simulink model "MdBsyClear4s"  (R2018b)
settings: Solver=FixedStepDiscrete  StartTime=0.0  StopTime=10.0  FixedStep=0.01  RelTol=1e-3
undefined symbols (not defined in the file or in its folder): ClearBit, IsStBsy32_Clear
settings Model: ModifiedHistory=2023.8.1 V2.0.0 CR401790 增加模式21-26  Creator=sn2xws  LastModifiedBy=sn2xws
settings DataIOCC: SaveFormat=StructureWithTime
settings OptimizationCC: DefaultParameterBehavior=Inlined  EnhancedBackFolding=on  PassReuseOutputArgsAs=Individual arguments  ZeroExternalMemoryAtStartup=off  ZeroInternalMemoryAtStartup=off  OptimizeBlockOrder=speed  DifferentSizesBufferReuse=on  OptimizationCustomize=off
settings DebuggingCC: ParameterTunabilityLossMsg=error
settings ModelReferenceCC: ModelReferenceNumInstancesAllowed=Single
settings SFSimCC: MATLABDynamicMemAlloc=off
settings RTWCC: SystemTargetFile=autosar.tlc  GenCodeOnly=on  TemplateMakefile=ert_default_tmf  Description=AUTOSAR  GenerateReport=on  IncludeHyperlinkInReport=on  LaunchReport=on  GenerateTraceInfo=on  GenerateTraceReport=on  GenerateTraceReportSl=on  GenerateTraceReportSf=on  GenerateTraceReportEml=on  GenerateCodeMetricsReport=on
settings CodeAppCC: ForceParamTrailComments=on  IgnoreCustomStorageClasses=off  OperatorAnnotations=on  SimulinkDataObjDesc=on  SFDataObjDesc=on  InsertBlockDesc=on
settings STFCustomTargetCC: TargetLangStandard=C99 (ISO)  MultiwordLength=256  ParMdlRefBuildCompliant=on  CompOptLevelCompliant=on  IncludeMdlTerminateFcn=off  CombineOutputUpdateFcns=on  SuppressErrorStatus=on  ERTCustomFileBanners=on  SupportNonFinite=off  SupportComplex=off  SupportContinuousTime=off  SupportNonInlinedSFcns=off  RemoveResetFunc=on  MATLABClassNameForMDSCustomization=Simulink.SoftwareTarget.ERTCustomization  AutosarCompliant=on  UseToolchainInfoCompliant=on  LookupTableObjectStructAxisOrder=2,1,3,4,...  LUTObjectStructOrderEvenSpacing=Size,Table,Breakpoints  SystemTargetFile=autosar.tlc
settings ERTTargetCC: TargetLangStandard=C99 (ISO)  ConcurrentExecutionCompliant=off  IncludeMdlTerminateFcn=off  SuppressErrorStatus=on  SupportNonFinite=off  SupportComplex=off  ModelStepFunctionPrototypeControlCompliant=off  CPPClassGenCompliant=off  AutosarCompliant=on  LookupTableObjectStructAxisOrder=2,1,3,4,...  LUTObjectStructOrderEvenSpacing=Size,Table,Breakpoints  InlinedParameterPlacement=NonHierarchical  ERTCustomFileTemplate=example_file_process.tlc  ERTFilePackagingFormat=Compact

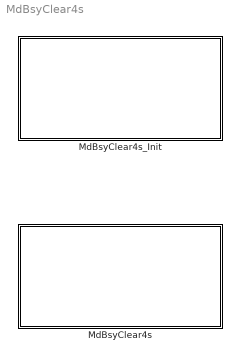
== system MdBsyClear4s ==
  MdBsyClear4s : Subsystem
  MdBsyClear4s_Init : Subsystem

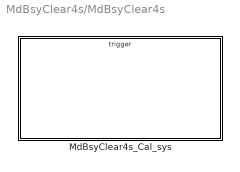
== system MdBsyClear4s/MdBsyClear4s ==
  MdBsyClear4s_Cal_sys : Subsystem

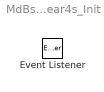
== system MdBsyClear4s/MdBsyClear4s_Init ==
  Event Listener : EventListener  EventName=reset

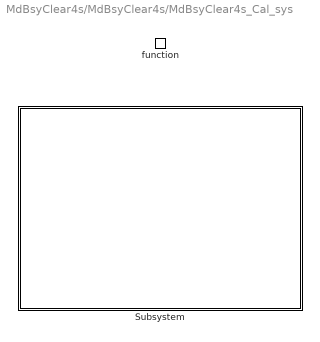
== system MdBsyClear4s/MdBsyClear4s/MdBsyClear4s_Cal_sys ==
  function : TriggerPort  TriggerType=function-call  IsSimulinkFunction=on  FunctionName=MdBsyClear4s_Cal  VariantControl=(inherit)
  Subsystem : Subsystem

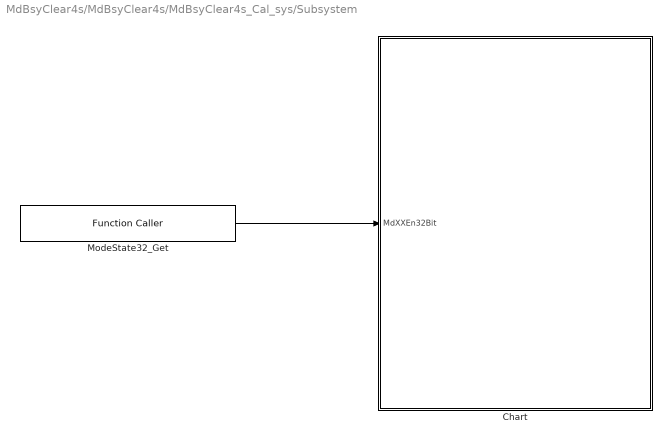
== system MdBsyClear4s/MdBsyClear4s/MdBsyClear4s_Cal_sys/Subsystem ==
  Chart : Stateflow chart  TreatAsAtomicUnit=on
  ModeState32_Get : FunctionCaller  FunctionPrototype=MdEn32 = ModeState32_Get()  OutputArgumentSpecifications=uint32(1)
  wires:
  ModeState32_Get/1 -> Chart/1(MdXXEn32Bit)

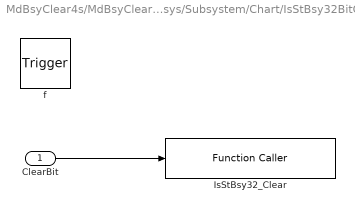
== system MdBsyClear4s/MdBsyClear4s/MdBsyClear4s_Cal_sys/Subsystem/Chart/IsStBsy32BitClear ==
  ClearBit : Inport
  f : TriggerPort  TriggerType=function-call  VariantControl=(inherit)
      settings: CopyFcn=Stateflow.SLINSF.SimulinkMan.removeBlockPreDeleteFcn  PreDeleteFcn=Stateflow.SLINSF.SimulinkMan.unsafePredeleteFcn
  IsStBsy32_Clear : FunctionCaller  FunctionPrototype=IsStBsy32_Clear(ClearBit)  InputArgumentSpecifications=uint32(1)
  wires:
  ClearBit/1 -> IsStBsy32_Clear/1

== stateflow chart MdBsyClear4s/MdBsyClear4s_Cal_sys/Subsystem/Chart ==
  state IsStBsy32BitClear(ClearBit) [function]
  note: 2023.8.1 V2.0.0 CR401790 增加模式21-26
  (default) -> (junction 17) : {
      | ClearBit = 0;
      | }
  (junction 17) -> (junction 43) [order 1] : [MdXXEn32Bit == 0]
  (junction 17) -> (junction 18) [order 2]
  (junction 43) -> (junction 45) : {ClearBit = (4294967295);}
  (junction 18) -> (junction 4) [order 1] : [((MdXXEn32Bit&LftMdBit4s) == 0)&&...
      | ((MdXXEn32Bit&WelcomeFwdBit) == 0)&&...
      | ((MdXXEn32Bit&WelcomeBkwdBit) == 0)]//LftMdBit4s=VIPL(2^9)+RecvyL(2^10)+LyL(2^13)+LgrstClsL(2^16)+LgrstOpenL(2^15)+EZE4sL(2^20)+EZQ4sL(2^21)=3253760
  (junction 18) -> (junction 15) [order 2]
  (junction 4) -> (junction 19) : {
      | ClearBit =(LftMdBit4s);
      | }
  (junction 19) -> (junction 15)
  (junction 15) -> (junction 7)
  (junction 7) -> (junction 21) [order 1] : [ ((MdXXEn32Bit&RghtMdBit4s) == 0)&&...
      | ((MdXXEn32Bit&WelcomeFwdBit) == 0)&&...
      | ((MdXXEn32Bit&WelcomeBkwdBit) == 0)]//RghtMdBit4s =VIPR(2^11)+RecvyR(2^12)+LyR(2^15)+LgrstClsR(2^18)+LgrstOpenR(2^17)+EZE4sR(2^22)+EZQ4sR(2^23)=13015040
  (junction 7) -> (junction 2) [order 2]
  (junction 21) -> (junction 6) : {
      | ClearBit =  (RghtMdBit4s);
      | }
  (junction 6) -> (junction 2)
  (junction 45) -> (junction 6)
  (junction 2) -> (junction 35) : {
      | IsStBsy32BitClear(ClearBit);
      | }
  data: ClearBit function_input; LftMdBit4s constant uint32 =3253760; RghtMdBit4s constant uint32 =13015040; MdXXEn32Bit input uint32; ClearBit local uint32; WelcomeFwdBit constant uint32 =16777216; WelcomeBkwdBit constant uint32 =33554432
